simulink model "simulinkSampledInput"  (R2017a)
settings: Solver=VariableStepAuto  StartTime=0.0  StopTime=30  RelTol=1e-3  EnableMultiTasking=on
values from neighbouring files (symbols this model uses):
  A = combPoly.A.polytopicMatrices{i}    [simulatesSampledInput.m]    (also in sin_simulatesSampledInput.m)
  B = [B1 B2]    [simulatesSampledInput.m]    (also in sin_simulatesSampledInput.m)
  C = combPoly.C.polytopicMatrices{i}    [simulatesSampledInput.m]    (also in sin_simulatesSampledInput.m)
  D1 = combPoly.D1.polytopicMatrices{i}    [simulatesSampledInput.m]    (also in sin_simulatesSampledInput.m)
  D2 = combPoly.D2.polytopicMatrices{i}    [simulatesSampledInput.m]    (also in sin_simulatesSampledInput.m)
undefined symbols (not defined in the file or in its folder): h, K
settings Model: Creator=1513 IRON  LastModifiedBy=Rafael
settings OptimizationCC: LifeSpan=inf
settings DebuggingCC: SFUnexpectedBacktrackingDiag=warning  SFNoUnconditionalDefaultTransitionDiag=warning  SFExecutionAtInitializationDiag=none
settings GRTTargetCC: TargetLangStandard=C89/C90 (ANSI)  GeneratePreprocessorConditionals=Disable all
settings ConfigComp: CovMetricSettings=dw  CovHtmlReporting=on  CovSaveCumulativeToWorkspaceVar=on  CovSaveSingleToWorkspaceVar=on  CovExternalEMLEnable=off

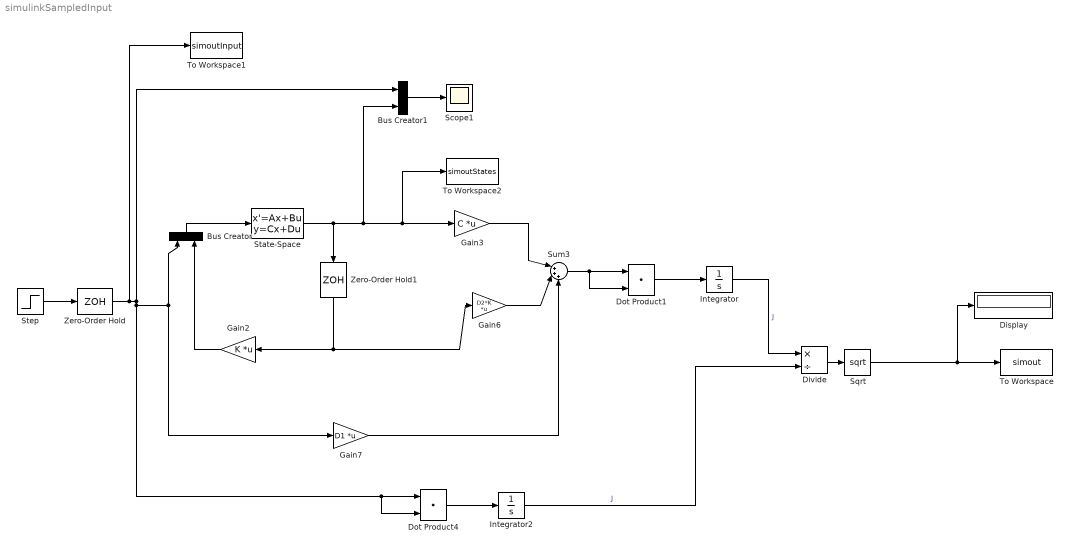
== system simulinkSampledInput ==
  Bus Creator : BusCreator  Inputs=2
  Bus Creator1 : BusCreator  Inputs=2
  Display : Display
  Divide : Product  Inputs=*/
  Dot Product1 : DotProduct  InputSameDT=on  OutDataTypeStr=Inherit: Inherit via internal rule
  Dot Product4 : DotProduct  InputSameDT=on  OutDataTypeStr=Inherit: Inherit via internal rule
  Gain2 : Gain  Gain=K  Multiplication=Matrix(K*u)
  Gain3 : Gain  Gain=C  Multiplication=Matrix(K*u)
  Gain6 : Gain  Gain=D2*K  Multiplication=Matrix(K*u)
  Gain7 : Gain  Gain=D1  Multiplication=Matrix(K*u)
  Integrator : Integrator
  Integrator2 : Integrator
  Scope1 : Scope
  Sqrt : Sqrt  SaturateOnIntegerOverflow=on
  State-Space : StateSpace  A=A  B=B  C=eye(size(A,1))  D=zeros(size(A,1),size(B,2))  X0=zeros(length(A),1)
  Step : Step  Before=1  After=0  SampleTime=h
  Sum3 : Sum  Inputs=|+++
  To Workspace : ToWorkspace  VariableName=simout  SaveFormat=Timeseries  SampleTime=h/30
  To Workspace1 : ToWorkspace  VariableName=simoutInput  SaveFormat=Timeseries  SampleTime=h/30
  To Workspace2 : ToWorkspace  VariableName=simoutStates  SaveFormat=Timeseries  SampleTime=h/30
  Zero-Order Hold : ZeroOrderHold  SampleTime=h
  Zero-Order Hold1 : ZeroOrderHold  SampleTime=h
  wires:
  Integrator/1 -> Divide/1  "J"
  State-Space/1 -> To Workspace2/1, Gain3/1, Bus Creator1/2, Zero-Order Hold1/1
  Bus Creator/1 -> State-Space/1
  Step/1 -> Zero-Order Hold/1
  Gain3/1 -> Sum3/1
  Gain6/1 -> Sum3/2
  Sum3/1 -> Dot Product1/2, Dot Product1/1
  Gain7/1 -> Sum3/3
  Dot Product1/1 -> Integrator/1
  Zero-Order Hold/1 -> To Workspace1/1, Bus Creator/1, Gain7/1, Dot Product4/2, Dot Product4/1, Bus Creator1/1
  Dot Product4/1 -> Integrator2/1
  Integrator2/1 -> Divide/2  "J"
  Bus Creator1/1 -> Scope1/1
  Divide/1 -> Sqrt/1
  Sqrt/1 -> Display/1, To Workspace/1
  Zero-Order Hold1/1 -> Gain6/1, Gain2/1
  Gain2/1 -> Bus Creator/2
